simulink model "TWmethod"  (R2016b)
settings: Solver=VariableStepAuto  StartTime=0.0  StopTime=0.15  RelTol=1e-3
libraries: powerlib x18
(part 2 of 2)

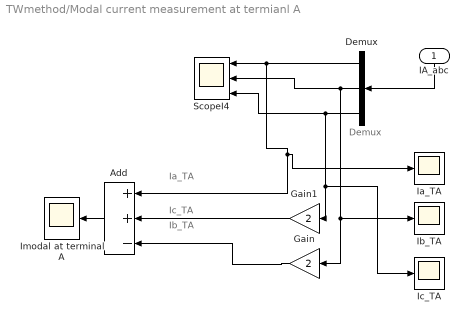
== system TWmethod/Modal current measurement at termianl A ==
  note: Ib_TA
  note: Ia_TA
  note: Ic_TA
  note: Demux
  IA_abc : Inport
  Add : Sum  Inputs=++-
  Demux : Demux  Outputs=3
  Gain : Gain  Gain=2
  Gain1 : Gain  Gain=2
  Ia_TA : Scope
  Ib_TA : Scope
  Ic_TA : Scope
  Imodal at terminal A : Scope
  ScopeI4 : Scope  NumInputPorts=3
  wires:
  Demux/1 -> Ia_TA/1, Add/1, ScopeI4/1
  Demux/2 -> Ib_TA/1, Gain/1, ScopeI4/2
  Demux/3 -> Ic_TA/1, Gain1/1, ScopeI4/3
  Gain1/1 -> Add/2
  Gain/1 -> Add/3
  Add/1 -> Imodal at terminal A/1
  IA_abc/1 -> Demux/1

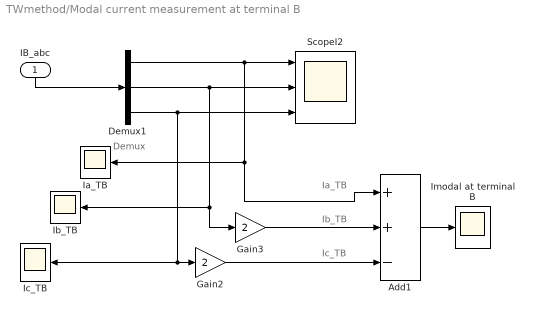
== system TWmethod/Modal current measurement at terminal B ==
  note: Ic_TB
  note: Ib_TB
  note: Ia_TB
  note: Demux
  IB_abc : Inport
  Add1 : Sum  Inputs=++-
  Demux1 : Demux  Outputs=3
  Gain2 : Gain  Gain=2
  Gain3 : Gain  Gain=2
  Ia_TB : Scope
  Ib_TB : Scope
  Ic_TB : Scope
  Imodal at terminal B : Scope
  ScopeI2 : Scope  NumInputPorts=3
  wires:
  Demux1/1 -> Add1/1, Ia_TB/1, ScopeI2/1
  Demux1/3 -> Ic_TB/1, Gain2/1, ScopeI2/3
  Gain3/1 -> Add1/2
  Demux1/2 -> Ib_TB/1, Gain3/1, ScopeI2/2
  Gain2/1 -> Add1/3
  Add1/1 -> Imodal at terminal B/1
  IB_abc/1 -> Demux1/1
